simulink model "ICCNetwork9_2_nf_EGM3_p1"  (R2018b)
settings: Solver=ode1  StartTime=0.0  StopTime=200  FixedStep=0.001  RelTol=1e-3
libraries: icc_lib_avg_path1_n1 x42
settings Model: PauseTimes=44.015  SnapshotBufferSize=100  Creator=lwan353  LastModifiedBy=lwan353
settings DebuggingCC: UnderSpecifiedDimensionMsg=warning
settings SFSimCC: SimUseLocalCustomCode=off
settings RTWCC: RTWUseLocalCustomCode=off

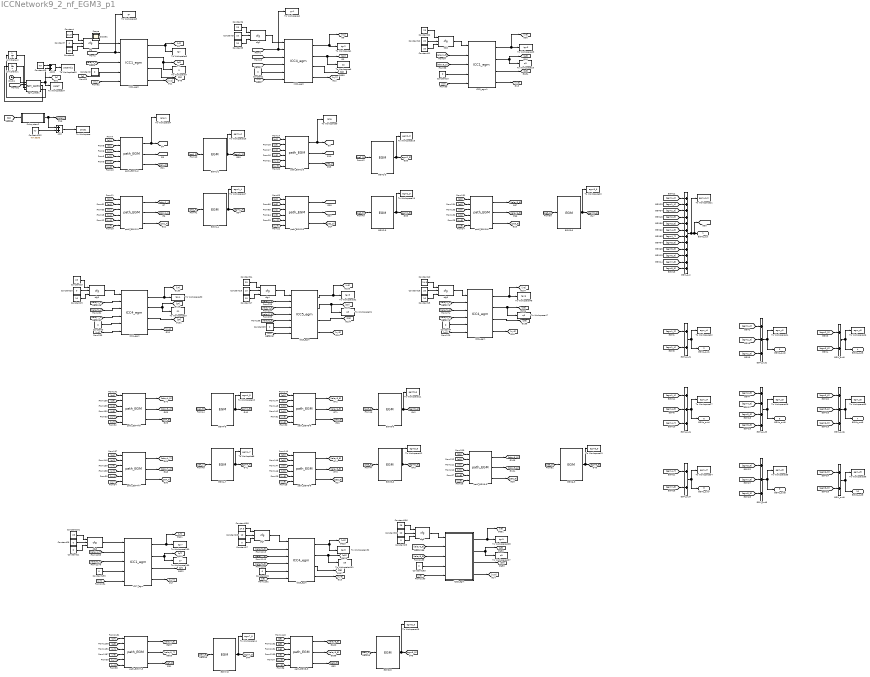
== system ICCNetwork9_2_nf_EGM3_p1 ==
  Add : Sum
  Add2 : Sum
  Clock1 : Clock
  Constant : Constant  Value=21.5
  Constant{1..4,7,10,20..21,25..27,29,182..183,193} (15 alike) : Constant  Value=0
  Constant{5,8,11..12,16,30} (6 alike) : Constant  Value=20
  Constant13 : Constant  Value=-67
  Constant{9,15,17..19,28} (6 alike) : Constant  Value=10
  Constant{6,22..24,181} (5 alike) : Constant  Value=23
  Constant196 : Constant  Value=26
  Constant198 : Constant  Value=24.5
  Constant202 : Constant  Value=-67.6336
  Constant40 : Constant  Value=24.5
  EGM1-2 : icc_lib_avg_path1_n1/EGM  SystemSampleTime=-1
  EGM1-4 : icc_lib_avg_path1_n1/EGM  SystemSampleTime=-1
  EGM2-3 : icc_lib_avg_path1_n1/EGM  SystemSampleTime=-1
  EGM2-5 : icc_lib_avg_path1_n1/EGM  SystemSampleTime=-1
  EGM3-6 : icc_lib_avg_path1_n1/EGM  SystemSampleTime=-1
  EGM4-5 : icc_lib_avg_path1_n1/EGM  SystemSampleTime=-1
  EGM4-7 : icc_lib_avg_path1_n1/EGM  SystemSampleTime=-1
  EGM5-6 : icc_lib_avg_path1_n1/EGM  SystemSampleTime=-1
  EGM5-8 : icc_lib_avg_path1_n1/EGM  SystemSampleTime=-1
  EGM6-9 : icc_lib_avg_path1_n1/EGM  SystemSampleTime=-1
  EGM7-8 : icc_lib_avg_path1_n1/EGM  SystemSampleTime=-1
  EGM8-9 : icc_lib_avg_path1_n1/EGM  SystemSampleTime=-1
  EGM_out : Sum  Inputs=12
  EGM_out{1,3,7,9} (4 alike) : Sum  Inputs=2
  EGM_out{2,4,6,8} (4 alike) : Sum  Inputs=3
  EGM_out5 : Sum  Inputs=4
  ICC1_egm : icc_lib_avg_path1_n1/ICC1_egm  SystemSampleTime=-1
  ICC2_egm : icc_lib_avg_path1_n1/ICC4_egm  SystemSampleTime=-1
  ICC3_egm1 : icc_lib_avg_path1_n1/ICC1_egm  SystemSampleTime=-1
  ICC4_egm : icc_lib_avg_path1_n1/ICC4_egm  SystemSampleTime=-1
  ICC5_egm : icc_lib_avg_path1_n1/ICC5_egm  SystemSampleTime=-1
  ICC6_egm : icc_lib_avg_path1_n1/ICC4_egm  SystemSampleTime=-1
  ICC7_egm : icc_lib_avg_path1_n1/ICC1_egm  SystemSampleTime=-1
  ICC8_egm : icc_lib_avg_path1_n1/ICC4_egm  SystemSampleTime=-1
  ICC9_egm : Subsystem  AncestorBlock=icc_lib_avg_path1_n1/ICC1_egm
  Subsystem2 : Subsystem  AncestorBlock=Pacemaker/Subsystem
  To Workspace : ToWorkspace  VariableName=pace1  SaveFormat=Timeseries  SampleTime=-1
  To Workspace1 : ToWorkspace  VariableName=tgv2  SaveFormat=Timeseries  SampleTime=-1
  To Workspace10 : ToWorkspace  VariableName=egm4_5  SaveFormat=Timeseries  SampleTime=-1
  To Workspace11 : ToWorkspace  VariableName=egm5_6  SaveFormat=Timeseries  SampleTime=-1
  To Workspace12 : ToWorkspace  VariableName=egm5_8  SaveFormat=Timeseries  SampleTime=-1
  To Workspace13 : ToWorkspace  VariableName=egm6_9  SaveFormat=Timeseries  SampleTime=-1
  To Workspace14 : ToWorkspace  VariableName=egm7_8  SaveFormat=Timeseries  SampleTime=-1
  To Workspace15 : ToWorkspace  VariableName=egm8_9  SaveFormat=Timeseries  SampleTime=-1
  To Workspace16 : ToWorkspace  VariableName=egm1_2  SaveFormat=Timeseries  SampleTime=-1
  To Workspace17 : ToWorkspace  VariableName=egm1_4  SaveFormat=Timeseries  SampleTime=-1
  To Workspace18 : ToWorkspace  VariableName=egm2_3  SaveFormat=Timeseries  SampleTime=-1
  To Workspace189 : ToWorkspace  VariableName=q7  SaveFormat=Timeseries  SampleTime=-1
  To Workspace19 : ToWorkspace  VariableName=egm2_5  SaveFormat=Timeseries  SampleTime=-1
  To Workspace190 : ToWorkspace  VariableName=tgv7  SaveFormat=Timeseries  SampleTime=-1
  To Workspace191 : ToWorkspace  VariableName=q8  SaveFormat=Timeseries  SampleTime=-1
  To Workspace192 : ToWorkspace  VariableName=tgv8  SaveFormat=Timeseries  SampleTime=-1
  To Workspace2 : ToWorkspace  VariableName=gv1  SaveFormat=Timeseries  SampleTime=-1
  To Workspace20 : ToWorkspace  VariableName=egm3_6  SaveFormat=Timeseries  SampleTime=-1
  To Workspace207 : ToWorkspace  VariableName=q9  SaveFormat=Timeseries  SampleTime=-1
  To Workspace208 : ToWorkspace  VariableName=tgv9  SaveFormat=Timeseries  SampleTime=-1
  To Workspace21 : ToWorkspace  VariableName=egm_sum  SaveFormat=Timeseries  SampleTime=-1
  To Workspace22 : ToWorkspace  VariableName=egm_c1  SaveFormat=Timeseries  SampleTime=-1
  To Workspace23 : ToWorkspace  VariableName=tgv3  SaveFormat=Timeseries  SampleTime=-1
  To Workspace24 : ToWorkspace  VariableName=egm_c2  SaveFormat=Timeseries  SampleTime=-1
  To Workspace25 : ToWorkspace  VariableName=q3  SaveFormat=Timeseries  SampleTime=-1
  To Workspace26 : ToWorkspace  VariableName=egm_c3  SaveFormat=Timeseries  SampleTime=-1
  To Workspace27 : ToWorkspace  VariableName=egm_c4  SaveFormat=Timeseries  SampleTime=-1
  To Workspace28 : ToWorkspace  VariableName=egm_c5  SaveFormat=Timeseries  SampleTime=-1
  To Workspace29 : ToWorkspace  VariableName=q4  SaveFormat=Timeseries  SampleTime=-1
  To Workspace3 : ToWorkspace  VariableName=tgv  SaveFormat=Timeseries  SampleTime=-1
  To Workspace30 : ToWorkspace  VariableName=tgv4  SaveFormat=Timeseries  SampleTime=-1
  To Workspace31 : ToWorkspace  VariableName=q5  SaveFormat=Timeseries  SampleTime=-1
  To Workspace32 : ToWorkspace  VariableName=tgv5  SaveFormat=Timeseries  SampleTime=-1
  To Workspace33 : ToWorkspace  VariableName=egm_c6  SaveFormat=Timeseries  SampleTime=-1
  To Workspace34 : ToWorkspace  VariableName=egm_c7  SaveFormat=Timeseries  SampleTime=-1
  To Workspace35 : ToWorkspace  VariableName=egm_c8  SaveFormat=Timeseries  SampleTime=-1
  To Workspace36 : ToWorkspace  VariableName=egm_c9  SaveFormat=Timeseries  SampleTime=-1
  To Workspace37 : ToWorkspace  VariableName=paceT  SaveFormat=Timeseries  SampleTime=-1
  To Workspace38 : ToWorkspace  VariableName=paceAdj1  SaveFormat=Timeseries  SampleTime=-1
  To Workspace4 : ToWorkspace  VariableName=relay1  SaveFormat=Timeseries  SampleTime=-1
  To Workspace47 : ToWorkspace  VariableName=q6  SaveFormat=Timeseries  SampleTime=-1
  To Workspace48 : ToWorkspace  VariableName=tgv6  SaveFormat=Timeseries  SampleTime=-1
  To Workspace5 : ToWorkspace  VariableName=gv  SaveFormat=Timeseries  SampleTime=-1
  To Workspace6 : ToWorkspace  VariableName=q2  SaveFormat=Timeseries  SampleTime=-1
  To Workspace7 : ToWorkspace  VariableName=q  SaveFormat=Timeseries  SampleTime=-1
  To Workspace8 : ToWorkspace  VariableName=egm4_7  SaveFormat=Timeseries  SampleTime=-1
  To Workspace9 : ToWorkspace  VariableName=relay  SaveFormat=Timeseries  SampleTime=-1
  Unit Delay1 : UnitDelay  SampleTime=-1
  Unit Delay2 : UnitDelay  SampleTime=-1
  cfg{,1..8} (9 alike) : icc_lib_avg_path1_n1/cfg  SystemSampleTime=-1
  egm_pace1 : icc_lib_avg_path1_n1/egm_pace1  SystemSampleTime=-1
  path_EGM1-2 : icc_lib_avg_path1_n1/path_EGM  SystemSampleTime=-1
  path_EGM1-4 : icc_lib_avg_path1_n1/path_EGM  SystemSampleTime=-1
  path_EGM2-3 : icc_lib_avg_path1_n1/path_EGM  SystemSampleTime=-1
  path_EGM2-5 : icc_lib_avg_path1_n1/path_EGM  SystemSampleTime=-1
  path_EGM3-6 : icc_lib_avg_path1_n1/path_EGM  SystemSampleTime=-1
  path_EGM4-5 : icc_lib_avg_path1_n1/path_EGM  SystemSampleTime=-1
  path_EGM4-7 : icc_lib_avg_path1_n1/path_EGM  SystemSampleTime=-1
  path_EGM5-6 : icc_lib_avg_path1_n1/path_EGM  SystemSampleTime=-1
  path_EGM5-8 : icc_lib_avg_path1_n1/path_EGM  SystemSampleTime=-1
  path_EGM6-9 : icc_lib_avg_path1_n1/path_EGM  SystemSampleTime=-1
  path_EGM7-8 : icc_lib_avg_path1_n1/path_EGM  SystemSampleTime=-1
  path_EGM8-9 : icc_lib_avg_path1_n1/path_EGM  SystemSampleTime=-1
  EGMs_out : Outport
  EGMs_out1 : Outport  Port=2
  EGMs_out2 : Outport  Port=3
  EGMs_out3 : Outport  Port=4
  EGMs_out5 : Outport  Port=5
  EGMs_out4 : Outport  Port=6
  EGMs_out6 : Outport  Port=7
  EGMs_out7 : Outport  Port=8
  EGMs_out8 : Outport  Port=9
  EGMs_out9 : Outport  Port=10
  Scope : Scope
  Scope1 : Scope
  wires:
  cfg1/1 -> ICC2_egm/1
  ICC2_egm/1 -> [v2], To Workspace1/1
  Constant1/1 -> ICC2_egm/5
  [v2] -> ICC2_egm/6
  [relay1_2] -> ICC2_egm/2, To Workspace2/1
  [q1] -> path_EGM1-2/1
  [v2] -> path_EGM1-2/4
  ICC2_egm/2 -> To Workspace6/1, [q2]
  [v1] -> path_EGM1-2/3
  [q2] -> path_EGM1-2/2
  path_EGM1-2/1 -> To Workspace4/1, [relay1_2]
  path_EGM1-2/2 -> [relay2_1]
  path_EGM2-3/1 -> To Workspace9/1, [relay2_3]
  [q2] -> path_EGM2-3/1
  path_EGM2-3/2 -> [relay3_2]
  [v2] -> path_EGM2-3/3
  [q3] -> path_EGM2-3/2
  [v3] -> path_EGM2-3/4
  [relay3_2] -> ICC2_egm/3
  ICC3_egm1/2 -> [q3], To Workspace25/1
  [relay6_3] -> ICC3_egm1/3
  [relay2_3] -> ICC3_egm1/2
  Constant10/1 -> ICC3_egm1/4
  ICC3_egm1/1 -> [v3], To Workspace23/1
  [v3] -> ICC3_egm1/5
  [v4] -> path_EGM1-4/4
  [q1] -> path_EGM1-4/1
  [v1] -> path_EGM1-4/3
  path_EGM1-4/2 -> [relay4_1]
  [q4] -> path_EGM1-4/2
  path_EGM1-4/1 -> [relay1_4]
  cfg/1 -> ICC1_egm/1
  [relay4_1] -> ICC1_egm/3
  ICC1_egm/1 -> To Workspace3/1, [v1]
  [relay2_1] -> ICC1_egm/2, To Workspace5/1
  [p] -> ICC1_egm/4
  [v1] -> ICC1_egm/5
  ICC1_egm/2 -> To Workspace7/1, [q1]
  [v5] -> path_EGM2-5/4
  [q2] -> path_EGM2-5/1
  [v2] -> path_EGM2-5/3
  path_EGM2-5/2 -> [relay5_2]
  [q5] -> path_EGM2-5/2
  path_EGM2-5/1 -> [relay2_5]
  [relay5_2] -> ICC2_egm/4
  [S1] -> Subsystem2/1(Sense)
  ICC1_egm/3 -> [S1]
  Constant/1 -> cfg/1
  path_EGM3-6/2 -> [relay6_3]
  [q3] -> path_EGM3-6/1
  [v6] -> path_EGM3-6/4
  [q6] -> path_EGM3-6/2
  path_EGM3-6/1 -> [relay3_6]
  [v3] -> path_EGM3-6/3
  [v6] -> ICC6_egm/6
  Constant4/1 -> ICC6_egm/5
  [q4] -> path_EGM4-7/1
  [v7] -> path_EGM4-7/4
  [q7] -> path_EGM4-7/2
  [q4] -> path_EGM4-5/1
  [q5] -> path_EGM4-5/2
  [v4] -> path_EGM4-5/3
  [v5] -> path_EGM4-5/4
  path_EGM4-5/2 -> [relay5_4]
  [v4] -> path_EGM4-7/3
  path_EGM4-5/1 -> [relay4_5]
  [q5] -> path_EGM5-8/1
  [v8] -> path_EGM5-8/4
  [q8] -> path_EGM5-8/2
  [q5] -> path_EGM5-6/1
  [q6] -> path_EGM5-6/2
  [v5] -> path_EGM5-6/3
  [v6] -> path_EGM5-6/4
  [v5] -> path_EGM5-8/3
  [q6] -> path_EGM6-9/1
  [v9] -> path_EGM6-9/4
  [v6] -> path_EGM6-9/3
  [q9] -> path_EGM6-9/2
  Constant6/1 -> cfg1/1
  cfg2/1 -> ICC3_egm1/1
  Constant22/1 -> cfg2/1
  [relay7_4] -> ICC4_egm/4
  [relay1_4] -> ICC4_egm/2
  cfg3/1 -> ICC4_egm/1
  Constant23/1 -> cfg3/1
  [relay5_4] -> ICC4_egm/3
  Constant3/1 -> ICC4_egm/5
  [v4] -> ICC4_egm/6
  ICC4_egm/1 -> [v4], To Workspace30/1
  ICC4_egm/2 -> [q4], To Workspace29/1
  ICC4_egm/3 -> [S4]
  ICC5_egm/1 -> [v5], To Workspace32/1
  ICC5_egm/2 -> To Workspace31/1, [q5]
  ICC5_egm/3 -> [S5]
  ICC6_egm/1 -> [v6], To Workspace48/1
  ICC6_egm/2 -> To Workspace47/1, [q6]
  ICC6_egm/3 -> [S6]
  [relay6_5] -> ICC5_egm/4
  [relay4_5] -> ICC5_egm/3
  [relay8_5] -> ICC5_egm/5
  cfg4/1 -> ICC5_egm/1
  Constant25/1 -> ICC5_egm/6
  [v5] -> ICC5_egm/7
  Constant24/1 -> cfg4/1
  [relay2_5] -> ICC5_egm/2
  [relay3_6] -> ICC6_egm/2
  [relay5_6] -> ICC6_egm/3
  [relay9_6] -> ICC6_egm/4
  cfg5/1 -> ICC6_egm/1
  Constant40/1 -> cfg5/1
  path_EGM4-7/1 -> [relay4_7]
  path_EGM4-7/2 -> [relay7_4]
  path_EGM5-6/1 -> [relay5_6]
  path_EGM5-6/2 -> [relay6_5]
  path_EGM5-8/1 -> [relay5_8]
  path_EGM5-8/2 -> [relay8_5]
  path_EGM6-9/1 -> [relay6_9]
  path_EGM6-9/2 -> [relay9_6]
  [v8] -> path_EGM7-8/4
  [relay8_7] -> ICC7_egm/3
  cfg8/1 -> ICC7_egm/1
  [relay9_8] -> ICC8_egm/4
  [relay7_8] -> ICC8_egm/3
  path_EGM7-8/1 -> [relay7_8]
  [q8] -> path_EGM7-8/2
  [relay6_9] -> ICC9_egm/2(gv1)
  [v7] -> ICC7_egm/5
  Constant193/1 -> ICC7_egm/4
  [relay8_9] -> ICC9_egm/3(gv2)
  Constant183/1 -> ICC9_egm/4(pulse)
  [relay4_7] -> ICC7_egm/2
  [v8] -> path_EGM8-9/3
  Constant196/1 -> cfg6/1
  [q8] -> path_EGM8-9/1
  path_EGM7-8/2 -> [relay8_7]
  [v9] -> path_EGM8-9/4
  [q9] -> path_EGM8-9/2
  [relay5_8] -> ICC8_egm/2
  Constant181/1 -> cfg8/1
  [v7] -> path_EGM7-8/3
  [q7] -> path_EGM7-8/1
  Constant182/1 -> ICC8_egm/5
  [v9] -> ICC9_egm/5(vin)
  cfg7/1 -> ICC8_egm/1
  cfg6/1 -> ICC9_egm/1("cfg ")
  Constant198/1 -> cfg7/1
  [v8] -> ICC8_egm/6
  ICC7_egm/3 -> [S7]
  ICC7_egm/2 -> [q7], To Workspace189/1
  ICC7_egm/1 -> [v7], To Workspace190/1
  ICC8_egm/2 -> To Workspace191/1, [q8]
  ICC8_egm/1 -> [v8], To Workspace192/1
  ICC9_egm/3(Output) -> [S9]
  ICC9_egm/2(q) -> [q9], To Workspace207/1
  ICC9_egm/1(v) -> [v9], To Workspace208/1
  ICC3_egm1/3 -> [S3]
  ICC2_egm/3 -> [S2]
  path_EGM8-9/1 -> [relay8_9]
  path_EGM8-9/2 -> [relay9_8]
  ICC8_egm/3 -> [S8]
  Add/1 -> To Workspace/1
  Constant202/1 -> Add/2
  Subsystem2/1(pace) -> Add/1, [pace1]
  Constant5/1 -> cfg/3
  Constant7/1 -> cfg/2
  Constant8/1 -> cfg1/3
  Constant9/1 -> cfg1/2
  Constant11/1 -> cfg2/3
  Constant12/1 -> cfg2/2
  Constant15/1 -> cfg5/3
  Constant16/1 -> cfg5/2
  Constant17/1 -> cfg4/3
  Constant18/1 -> cfg4/2
  Constant19/1 -> cfg3/3
  Constant20/1 -> cfg3/2
  Constant21/1 -> cfg8/3
  Constant26/1 -> cfg8/2
  Constant27/1 -> cfg7/3
  Constant28/1 -> cfg7/2
  Constant29/1 -> cfg6/3
  Constant30/1 -> cfg6/2
  ICC1_egm/4 -> [xy1]
  ICC2_egm/4 -> [xy2]
  ICC3_egm1/4 -> [xy3]
  ICC9_egm/4(xy) -> [xy9]
  ICC8_egm/4 -> [xy8]
  ICC7_egm/4 -> [xy7]
  ICC6_egm/4 -> [xy6]
  ICC5_egm/4 -> [xy5]
  ICC4_egm/4 -> [xy4]
  [xy1] -> path_EGM1-2/5
  [xy2] -> path_EGM1-2/6
  [xy1] -> path_EGM1-4/5
  [xy4] -> path_EGM1-4/6
  [xy3] -> path_EGM2-3/6
  [xy2] -> path_EGM2-3/5
  [xy5] -> path_EGM2-5/6
  [xy2] -> path_EGM2-5/5
  [xy6] -> path_EGM3-6/6
  [xy3] -> path_EGM3-6/5
  [xy9] -> path_EGM6-9/6
  [xy6] -> path_EGM6-9/5
  [xy8] -> path_EGM5-8/6
  [xy5] -> path_EGM5-8/5
  [xy6] -> path_EGM5-6/6
  [xy5] -> path_EGM5-6/5
  [xy5] -> path_EGM4-5/6
  [xy4] -> path_EGM4-5/5
  [xy7] -> path_EGM4-7/6
  [xy4] -> path_EGM4-7/5
  [xy9] -> path_EGM8-9/6
  [xy8] -> path_EGM8-9/5
  [xy8] -> path_EGM7-8/6
  [xy7] -> path_EGM7-8/5
  path_EGM1-2/3 -> [pe1_2]
  path_EGM1-4/3 -> [pe1_4]
  path_EGM2-3/3 -> [pe2_3]
  path_EGM2-5/3 -> [pe2_5]
  path_EGM3-6/3 -> [pe3_6]
  path_EGM5-6/3 -> [pe5_6]
  path_EGM5-8/3 -> [pe5_8]
  path_EGM6-9/3 -> [pe6_9]
  path_EGM4-5/3 -> [pe4_5]
  path_EGM4-7/3 -> [pe4_7]
  path_EGM7-8/3 -> [pe7_8]
  path_EGM8-9/3 -> [pe8_9]
  [pe1_2] -> EGM1-2/1
  [pe1_4] -> EGM1-4/1
  EGM1-2/1 -> To Workspace16/1, [egm1_2]
  EGM1-4/1 -> To Workspace17/1, [egm1_4]
  [pe2_3] -> EGM2-3/1
  EGM2-3/1 -> To Workspace18/1, [egm2_3]
  [pe2_5] -> EGM2-5/1
  EGM2-5/1 -> To Workspace19/1, [egm2_5]
  [pe4_5] -> EGM4-5/1
  EGM4-5/1 -> To Workspace10/1, [egm4_5]
  [pe4_7] -> EGM4-7/1
  EGM4-7/1 -> [egm4_7], To Workspace8/1
  [pe5_6] -> EGM5-6/1
  EGM5-6/1 -> [egm5_6], To Workspace11/1
  [pe5_8] -> EGM5-8/1
  EGM5-8/1 -> To Workspace12/1, [egm5_8]
  [pe7_8] -> EGM7-8/1
  EGM7-8/1 -> To Workspace14/1, [egm7_8]
  [pe8_9] -> EGM8-9/1
  EGM8-9/1 -> To Workspace15/1, [egm8_9]
  [pe3_6] -> EGM3-6/1
  EGM3-6/1 -> To Workspace20/1, [egm3_6]
  [pe6_9] -> EGM6-9/1
  EGM6-9/1 -> To Workspace13/1, [egm6_9]
  [egm1_4] -> EGM_out/2
  EGM_out/1 -> To Workspace21/1, [egm_sum], EGMs_out/1
  [egm1_2] -> EGM_out/1
  [egm2_3] -> EGM_out/3
  [egm5_8] -> EGM_out/9
  [egm5_6] -> EGM_out/8
  [egm4_7] -> EGM_out/7
  [egm4_5] -> EGM_out/6
  [egm3_6] -> EGM_out/5
  [egm2_5] -> EGM_out/4
  [egm7_8] -> EGM_out/11
  [egm6_9] -> EGM_out/10
  [egm8_9] -> EGM_out/12
  EGM_out1/1 -> EGMs_out1/1, To Workspace22/1
  [egm1_4] -> EGM_out1/2
  [egm1_2] -> EGM_out1/1
  [egm2_5] -> EGM_out2/3
  [egm2_3] -> EGM_out2/2
  EGM_out2/1 -> EGMs_out2/1, To Workspace24/1
  [egm1_2] -> EGM_out2/1
  [egm3_6] -> EGM_out3/2
  EGM_out3/1 -> To Workspace26/1, EGMs_out3/1
  [egm2_3] -> EGM_out3/1
  [egm4_5] -> EGM_out5/2
  [egm5_6] -> EGM_out5/3
  EGM_out5/1 -> EGMs_out5/1, To Workspace28/1
  [egm2_5] -> EGM_out5/1
  [egm1_4] -> EGM_out4/1
  [egm4_7] -> EGM_out4/3
  EGM_out4/1 -> EGMs_out4/1, To Workspace27/1
  [egm4_5] -> EGM_out4/2
  [egm3_6] -> EGM_out6/1
  [egm6_9] -> EGM_out6/3
  EGM_out6/1 -> EGMs_out6/1, To Workspace33/1
  [egm5_6] -> EGM_out6/2
  [egm4_7] -> EGM_out7/1
  EGM_out7/1 -> EGMs_out7/1, To Workspace34/1
  [egm7_8] -> EGM_out8/2
  [egm8_9] -> EGM_out8/3
  EGM_out8/1 -> EGMs_out8/1, To Workspace35/1
  [egm5_8] -> EGM_out8/1
  [egm8_9] -> EGM_out9/2
  EGM_out9/1 -> EGMs_out9/1, To Workspace36/1
  [egm7_8] -> EGM_out7/2
  [egm6_9] -> EGM_out9/1
  [egm5_8] -> EGM_out5/4
  Add2/1 -> To Workspace38/1
  Unit Delay2/1 -> egm_pace1/4
  Constant13/1 -> Add2/1
  egm_pace1/3 -> Unit Delay2/1
  egm_pace1/1 -> Add2/2, To Workspace37/1, [p]
  egm_pace1/2 -> Unit Delay1/1
  [egm_sum] -> egm_pace1/2
  Clock1/1 -> egm_pace1/1
  Unit Delay1/1 -> egm_pace1/3

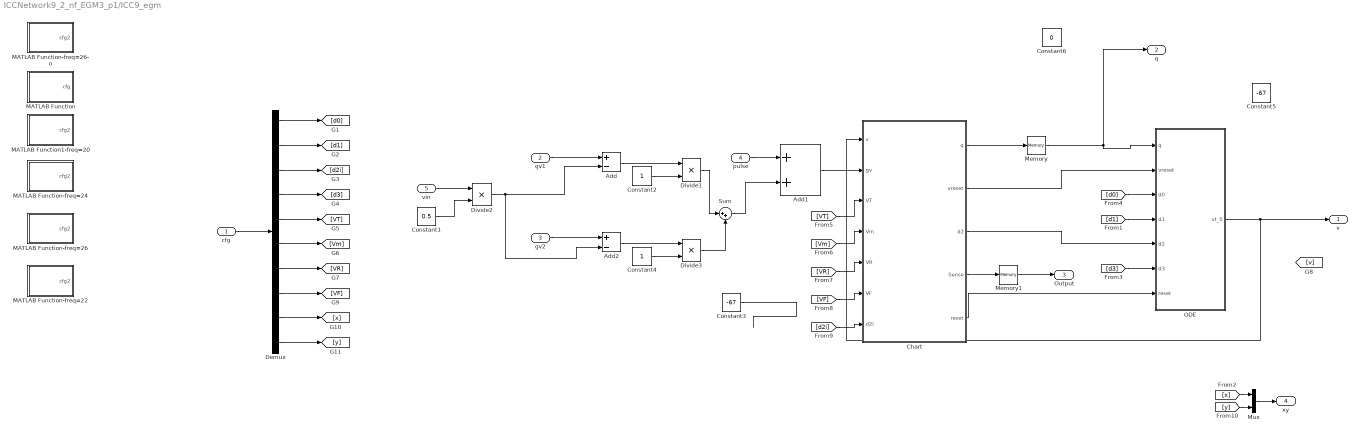
== system ICCNetwork9_2_nf_EGM3_p1/ICC9_egm ==
  "cfg " : Inport
  gv1 : Inport  Port=2
  gv2 : Inport  Port=3
  pulse : Inport  Port=4
  vin : Inport  Port=5
  Add : Sum  Inputs=+-
  Add1 : Sum
  Add2 : Sum  Inputs=+-
  Chart : Stateflow chart  TreatAsAtomicUnit=on
  Constant1 : Constant  Value=0.5
  Constant2 : Constant
  Constant3 : Constant  Value=-67
  Constant4 : Constant
  Constant5 : Constant  Value=-67
  Constant6 : Constant  Value=0
  Demux : Demux  Outputs=10
  Divide1 : Product  CollapseMode=Specified dimension  CollapseDim=2  SaturateOnIntegerOverflow=on  RndMeth=Zero
  Divide2 : Product  CollapseMode=Specified dimension  CollapseDim=2  SaturateOnIntegerOverflow=on  RndMeth=Zero
  Divide3 : Product  CollapseMode=Specified dimension  CollapseDim=2  SaturateOnIntegerOverflow=on  RndMeth=Zero
  MATLAB Function : MATLAB Function  TreatAsAtomicUnit=on
  "MATLAB Function-freq=22 " : MATLAB Function  TreatAsAtomicUnit=on
  MATLAB Function-freq=24 : MATLAB Function  TreatAsAtomicUnit=on
  "MATLAB Function-freq=26 " : MATLAB Function  TreatAsAtomicUnit=on
  "MATLAB Function-freq=26-o " : MATLAB Function  TreatAsAtomicUnit=on
  "MATLAB Function1-freq=20 " : MATLAB Function  TreatAsAtomicUnit=on
  Memory : Memory  InheritSampleTime=on
  Memory1 : Memory  InheritSampleTime=on
  Mux : Mux  Inputs=2
  ODE : Subsystem
  Sum : Sum  Inputs=|++
  v : Outport
  q : Outport  Port=2
  Output : Outport  Port=3
  xy : Outport  Port=4
  wires:
  [y] -> Mux/2
  [x] -> Mux/1
  Mux/1 -> xy/1
  Demux/10 -> [y]
  Demux/9 -> [x]
  Memory1/1 -> Output/1
  Chart/4(Sense) -> Memory1/1
  Sum/1 -> Add1/2
  Add2/1 -> Divide3/1
  Divide3/1 -> Sum/2
  Constant4/1 -> Divide3/2
  gv2/1 -> Add2/1
  Memory/1 -> q/1, ODE/1(q)
  Chart/1(q) -> Memory/1
  Constant3/1 -> ?
  Add/1 -> Divide1/1
  Divide2/1 -> Add/2, Add2/2
  Constant1/1 -> Divide2/2
  [d3] -> ODE/6(d3)
  Demux/6 -> [Vm]
  Demux/1 -> [d0]
  Demux/4 -> [d3]
  Chart/2(vreset) -> ODE/2(vreset)
  [d0] -> ODE/3(d0)
  Demux/7 -> [VR]
  Chart/3(d2) -> ODE/5(d2)
  [VT] -> Chart/3(VT)
  ODE/1(vt_0) -> Chart/1(v), v/1
  Demux/3 -> [d2i]
  [VR] -> Chart/5(VR)
  [VF] -> Chart/6(VF)
  [d2i] -> Chart/7(d2i)
  Demux/2 -> [d1]
  Add1/1 -> Chart/2(gv)
  Demux/5 -> [VT]
  "cfg "/1 -> Demux/1
  Chart/5(reset) -> ODE/7(reset)
  [Vm] -> Chart/4(Vm)
  [d1] -> ODE/4(d1)
  Demux/8 -> [VF]
  pulse/1 -> Add1/1
  Constant2/1 -> Divide1/2
  vin/1 -> Divide2/1
  Divide1/1 -> Sum/1
  gv1/1 -> Add/1

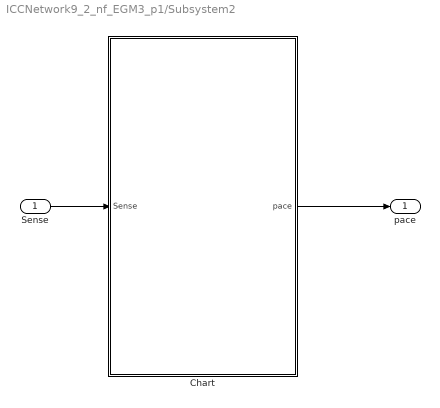
== system ICCNetwork9_2_nf_EGM3_p1/Subsystem2 ==
  Sense : Inport
  Chart : Stateflow chart  TreatAsAtomicUnit=on
  pace : Outport
  wires:
  Sense/1 -> Chart/1(Sense)
  Chart/1(pace) -> pace/1

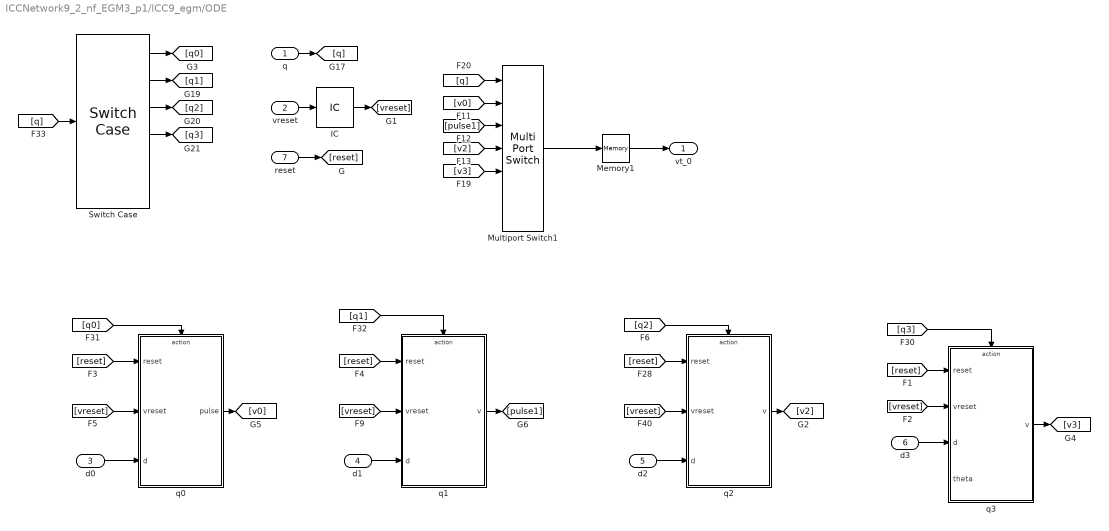
== system ICCNetwork9_2_nf_EGM3_p1/ICC9_egm/ODE ==
  q : Inport
  vreset : Inport  Port=2
  d0 : Inport  Port=3
  d1 : Inport  Port=4
  d2 : Inport  Port=5
  d3 : Inport  Port=6
  reset : Inport  Port=7
  IC : InitialCondition  Value=0
  Memory1 : Memory
  Multiport Switch1 : MultiPortSwitch  DataPortOrder=Zero-based contiguous  Inputs=6  zeroidx=on
  Switch Case : SwitchCase  CaseConditions={0,1,2,3,4,5}  ShowDefaultCase=off
  q0 : Subsystem  TreatAsAtomicUnit=on
  q1 : Subsystem  TreatAsAtomicUnit=on
  q2 : Subsystem  TreatAsAtomicUnit=on
  q3 : Subsystem  TreatAsAtomicUnit=on
  vt_0 : Outport
  wires:
  Multiport Switch1/1 -> Memory1/1
  IC/1 -> [vreset]
  vreset/1 -> IC/1
  reset/1 -> [reset]
  q/1 -> [q]
  q1/1(v) -> [pulse1]
  [q] -> Multiport Switch1/1
  [q] -> Switch Case/1
  [q1] -> q1/Action
  [reset] -> q1/1(reset)
  q2/1(v) -> [v2]
  d2/1 -> q2/3(d)
  [q2] -> q2/Action
  [vreset] -> q2/2(vreset)
  q3/1(v) -> [v3]
  d3/1 -> q3/3(d)
  [reset] -> q3/1(reset)
  [vreset] -> q3/2(vreset)
  q0/1(pulse) -> [v0]
  d0/1 -> q0/3(d)
  [reset] -> q0/1(reset)
  [vreset] -> q0/2(vreset)
  [q3] -> q3/Action
  [q0] -> q0/Action
  Memory1/1 -> vt_0/1
  [v0] -> Multiport Switch1/2
  [pulse1] -> Multiport Switch1/3
  [v2] -> Multiport Switch1/4
  [v3] -> Multiport Switch1/5
  [reset] -> q2/1(reset)
  [vreset] -> q1/2(vreset)
  d1/1 -> q1/3(d)
  Switch Case/1 -> [q0]
  Switch Case/2 -> [q1]
  Switch Case/3 -> [q2]
  Switch Case/4 -> [q3]

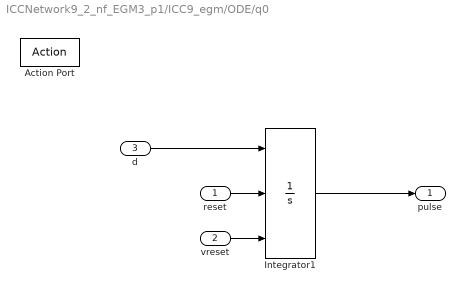
== system ICCNetwork9_2_nf_EGM3_p1/ICC9_egm/ODE/q0 ==
  reset : Inport
  vreset : Inport  Port=2
  d : Inport  Port=3
  Action Port : ActionPort  InitializeStates=reset  ActionType=case
  Integrator1 : Integrator  ExternalReset=either  InitialConditionSource=external  InitialCondition=20
  pulse : Outport
  wires:
  vreset/1 -> Integrator1/3
  reset/1 -> Integrator1/2
  d/1 -> Integrator1/1
  Integrator1/1 -> pulse/1

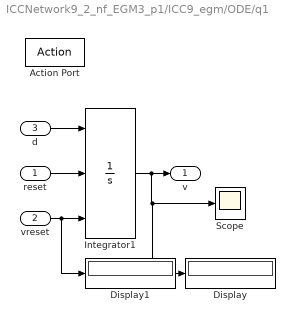
== system ICCNetwork9_2_nf_EGM3_p1/ICC9_egm/ODE/q1 ==
  reset : Inport
  vreset : Inport  Port=2
  d : Inport  Port=3
  Action Port : ActionPort  InitializeStates=reset  ActionType=case
  Display : Display
  Display1 : Display
  Integrator1 : Integrator  ExternalReset=either  InitialConditionSource=external  InitialCondition=20  LimitOutput=on  UpperSaturationLimit=-24.105
  Scope : Scope
  v : Outport
  wires:
  vreset/1 -> Integrator1/3, Display1/1
  reset/1 -> Integrator1/2
  Integrator1/1 -> v/1, Scope/1, Display/1
  d/1 -> Integrator1/1

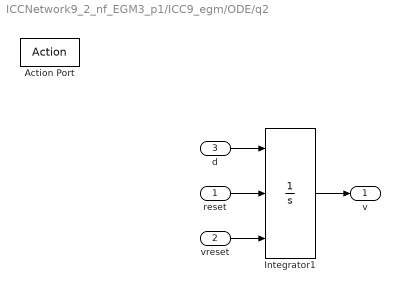
== system ICCNetwork9_2_nf_EGM3_p1/ICC9_egm/ODE/q2 ==
  reset : Inport
  vreset : Inport  Port=2
  d : Inport  Port=3
  Action Port : ActionPort  InitializeStates=reset  ActionType=case
  Integrator1 : Integrator  ExternalReset=either  InitialConditionSource=external  InitialCondition=20
  v : Outport
  wires:
  Integrator1/1 -> v/1
  reset/1 -> Integrator1/2
  vreset/1 -> Integrator1/3
  d/1 -> Integrator1/1

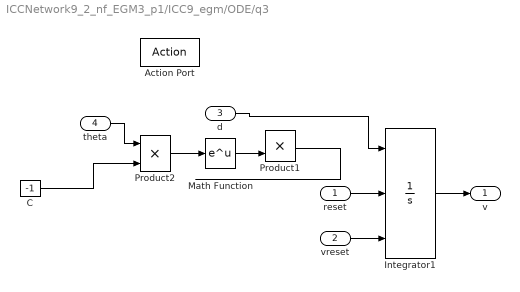
== system ICCNetwork9_2_nf_EGM3_p1/ICC9_egm/ODE/q3 ==
  reset : Inport
  vreset : Inport  Port=2
  d : Inport  Port=3
  theta : Inport  Port=4
  Action Port : ActionPort  InitializeStates=reset  ActionType=case
  C : Constant  Value=-1
  Integrator1 : Integrator  ExternalReset=either  InitialConditionSource=external  InitialCondition=20  LimitOutput=on  LowerSaturationLimit=-67
  Math Function : Math  SaturateOnIntegerOverflow=on
  Product1 : Product
  Product2 : Product
  v : Outport
  wires:
  vreset/1 -> Integrator1/3
  reset/1 -> Integrator1/2
  Integrator1/1 -> v/1
  Math Function/1 -> Product1/2
  theta/1 -> Product2/1
  Product1/1 -> ?
  C/1 -> Product2/2
  Product2/1 -> Math Function/1
  d/1 -> Integrator1/1

== stateflow chart ICCNetwork9_2_nf_EGM3_p1/Subsystem2/Chart ==
  state Pacemaker
    state GRP [parallel]
      settings: executionOrder=1
      state Idle
        du:
        sense=Sense;
      state StartGRP
        du:
        grp=1;
        Tgrp=temporalCount (sec);
      state EndGRP
        en:
        grp=0;
        endGRP=1;
      state Wait
      (default) -> Pacemaker.GRP.Idle : {grp=0;Tgrp=0;endGRP=0;sense=0;}
      Pacemaker.GRP.Idle -> StartGRP [order 1] : [sense==1&&grp==0]{sense=0;}
      StartGRP -> EndGRP : [Tgrp==5]{Tgrp=0;}
      Pacemaker.GRP.Idle -> Pacemaker.GRP.Wait [order 2] : [sense==1&&grp==1]{sense=0;}
      EndGRP -> Pacemaker.GRP.Idle
      Pacemaker.GRP.Wait -> Pacemaker.GRP.Idle
    state LRI [parallel]
      settings: executionOrder=2
      state EndLRI
        en:
        pace=2;
        du:
        s=Sense
      state StartLRI
        en:
        c = c +1;
        du:
        Tlri=temporalCount (sec);
      state Idle
        du:
        s=Sense;
      state wait
      state Wait
      state AfterGRPsense
      (default) -> Pacemaker.LRI.Idle : {Tlri=0;grp=0;endGRP=0;s=0;c=0;}
      StartLRI -> EndLRI [order 1] : [Tlri>=func3(c)]{Tlri=0}
      Pacemaker.LRI.Idle -> StartLRI [order 1] : [s==1&&grp==0]{s=0;}
      EndLRI -> StartLRI : [s==1]{pace=0;s=0;endGRP=0}
      Pacemaker.LRI.Wait -> Pacemaker.LRI.Idle
      Pacemaker.LRI.Idle -> Pacemaker.LRI.Wait [order 2] : [s==1&&grp==1]{s=0;}
      AfterGRPsense -> StartLRI
      StartLRI -> AfterGRPsense [order 3] : [endGRP==1&&Tlri<20&&sense==1]{Tlri=0;endGRP=0;s=0}
      wait -> StartLRI
      StartLRI -> wait [order 2] : [endGRP==0&&Tlri<20&&s==1]{sense=0;}
  (default) -> Pacemaker : {pace=0;}
  data: s local; c local; tlri function_output double; count function_input; pace output; Sense input; Tgrp local; Tlri local; grp local; endGRP local; sense local
  function tlri = func3(count):
    | function tlri = func3(count)
    | 
    | LRI=20;
    | offset=0;
    | %tlri=0;
    | if(count==1)
    |   tlri = LRI+offset;
    | 
    | %elseif(count>1)
    | else
    |   tlri = LRI;
    | 
    | end

== stateflow chart ICCNetwork9_2_nf_EGM3_p1/ICC9_egm/Chart ==
  state wait
    entry:
    du:
    t2=temporalCount (sec);
  state q0
    en:
    q=0
  state q1
    en:
    q=1
    Sense=1;
    exit:
    Sense=0;
  state q3
    en:
    q=3
  state q2
    en:
    q=2
  (default) -> wait : {t2=0;}
  wait -> q0 : [t2>=19.6]{q=0;vreset=-67.6336;reset}
  q0 -> q1 [order 1] : [v<VT]/{vreset=v;Vmax=Vm;d2=d2i;reset}
  q0 -> q1 [order 2] : [gv>VF&&v>VT]{ vreset=v; Vmax=Vm;d2=d2i;reset}
  q3 -> q0 : [v<VF]{vreset=v; reset}
  q1 -> q2 : [ v >Vmax ]{vreset=v; reset}
  q2 -> q3 : [v<VR]{vreset=v; reset}
  data: v input double; q output; vreset output; gv input double; VT input; Vm input; VR input; VF input; Vmax local; t2 local; d2i input; d2 output; Sense output
  events: reset output EITHER_EDGE_EVENT

== matlab function ICCNetwork9_2_nf_EGM3_p1/ICC9_egm/MATLAB Function ==
  data: cfg output
function cfg = fcn()

%d0-o= -0.039651515;
d0= -0.042051515;
d1= 216.5795;
d2= -0.7491129;
d3= -8.890176;
%d3-1= -8.960176;

VT= -67.6;
Vm= -24.3058;
VR= -28.9622;
VF= -66.9799;

cfg=[d0,d1,d2,d3,VT,Vm,VR,VF];

end

== matlab function ICCNetwork9_2_nf_EGM3_p1/ICC9_egm/MATLAB Function-freq=22  ==
  data: cfg2 output
function cfg2 = fcn()

%d0-o= -0.039651515;

%d0= -0.042051515;
%d1= 216.5795;
%d2= -0.7491129;
%d3= -8.890176;

%d3-1= -8.960176;

%freq=22
d0=-0.045;
d1=43.5373;
d2=-0.835;
d3=-6.96;


VT= -67.6336;
Vm= -24.1075;
VR= -28.8921;
VF= -66.9586;



cfg2=[d0,d1,d2,d3,VT,Vm,VR,VF];

end

== matlab function ICCNetwork9_2_nf_EGM3_p1/ICC9_egm/MATLAB Function-freq=24 ==
  data: cfg2 output
function cfg2 = fcn()

%d0-o= -0.039651515;

%d0= -0.042051515;
%d1= 216.5795;
%d2= -0.7491129;
%d3= -8.890176;

%d3-1= -8.960176;

%freq24
d0=-0.0381;
d1=43.568;
d2=-0.82;
d3=-4.8;


VT= -67.6336;
Vm= -24.1075;
VR= -28.8921;
VF= -66.9586;



cfg2=[d0,d1,d2,d3,VT,Vm,VR,VF];

end

== matlab function ICCNetwork9_2_nf_EGM3_p1/ICC9_egm/MATLAB Function-freq=26  ==
  data: cfg2 output
function cfg2 = fcn()

%d0-o= -0.039651515;

%d0= -0.042051515;
%d1= 216.5795;
%d2= -0.7491129;
%d3= -8.890176;

%d3-1= -8.960176;

%freq26
d0=-0.053;
d1=39.5735;
d2=-0.8035;
d3=-4.69678;


VT= -67.6336;
Vm= -24.1075;
VR= -28.8921;
VF= -66.9586;



cfg2=[d0,d1,d2,d3,VT,Vm,VR,VF];

end

== matlab function ICCNetwork9_2_nf_EGM3_p1/ICC9_egm/MATLAB Function-freq=26-o  ==
  data: cfg2 output
function cfg2 = fcn()

%d0-o= -0.039651515;

%d0= -0.042051515;
%d1= 216.5795;
%d2= -0.7491129;
%d3= -8.890176;

%d3-1= -8.960176;

%freq26
d0=-0.053;
d1=39.5735;
d2=-0.8035;
d3=-4.69678;


VT= -67.6336;
Vm= -24.1075;
VR= -28.8921;
VF= -66.9586;



cfg2=[d0,d1,d2,d3,VT,Vm,VR,VF];

end

== matlab function ICCNetwork9_2_nf_EGM3_p1/ICC9_egm/MATLAB Function1-freq=20  ==
  data: cfg2 output
function cfg2 = fcn()

%d0-o= -0.039651515;

%d0= -0.042051515;
%d1= 216.5795;
%d2= -0.7491129;
%d3= -8.890176;

%d3-1= -8.960176;


d0=-0.075;
d1=43.625;
d2=-0.88;
d3=-8.65;


VT= -67.6336;
Vm= -24.1075;
VR= -28.8921;
VF= -66.9586;



cfg2=[d0,d1,d2,d3,VT,Vm,VR,VF];

end
